simulink model "NMPC_BGLOSA_2VEH"  (R2022b)
settings: Solver=ode4  StartTime=0.0  StopTime=1500  FixedStep=0.1  RelTol=1e-3
PostLoadFcn:
  | , if any(exist('dsrtsu_mdlpostloadfcn', 'file') == [2, 3, 6]), try dsrtsu_mdlpostloadfcn('Execute', bdroot); catch fprintf('Error in PostLoadFcn (dsrtsu_mdlpostloadfcn) for model "%s":\n %s\n', bdroot, lasterr); end, end,
values from neighbouring files (symbols this model uses):
  k_road_map = k_road_map(:)    [NMPC_init_2veh.m]
  N = 50    [ACADO_2veh.m]    (also in NMPC_init_2veh.m; debug_vincoli_violati.m)
  N_iter = 3    [NMPC_init_2veh.m]
  N_Jterms = length(Qx1)    [NMPC_init_2veh.m]
  NMPC_Wmat1 = [W1(1,:) W1(2,:) W1(3,:) W1(4,:) W1(5,:) W1(6,:) W1(7,:) W1(8,:) W1(9,:) W1(10,:) W1(11,:) W1(12,:) W1(13,:) W1(14,:)]    [NMPC_init_2veh.m]
  NMPC_WNmat1 = reshape(WN1.',1,[])    [NMPC_init_2veh.m]
  t_dwell = 10    [ACADO_2veh.m]    (also in NMPC_init_2veh.m)
  t_offset = 0    [NMPC_init_2veh.m]
  time_bag_sim = (0:1:round(time_bag(end))-1)'    [NMPC_init_2veh.m]
  tl_state_sim = zeros(round(time_bag(end))-1,size(tl_col,2))    [NMPC_init_2veh.m]
  Ts = 1    [ACADO_2veh.m]    (also in NMPC_init_2veh.m)
  Vmax = 50    [NMPC_init_2veh.m]    (also in debug_vincoli_violati.m = OD(:,17))
  xInit = [20 2 0 0 1 0]    [NMPC_init_2veh.m]
undefined symbols (not defined in the file or in its folder): ds, s_start
libraries: simulink x1
(part 2 of 2)

== matlab function NMPC_BGLOSA_2VEH/NMPC WITH MOTOR DYNAMICS/ROAD PREVIEW/No ROAD PREVIEW ==
  data: x_TL input; stop_enabled input; Vmax input; Vmax_2 input; state_pred_old input; t_dwell input; time_cur input; reached_TL_old input; reached_TL_old_2 input; reached_stop_old input; reached_stop_old_2 input; t_piola_old input; t_loreto_old input; stop_dwell_count_old input; stop_dwell_count_old_2 input; OnlineData output; reached_TL output; reached_TL_2 output; reached_stop output; reached_stop_2 output; t_piola output; t_loreto output; debug_TL output; debug_TL_2 output; stop_dwell_count output; stop_dwell_count_2 output; red_stopline_hold output; s_hold output; k_road_hor input; red_stopline_hold2 output; s_hold2 output; k_road_hor_2 input
function [OnlineData, reached_TL, reached_TL_2, reached_stop, reached_stop_2, t_piola, t_loreto, debug_TL, debug_TL_2, stop_dwell_count, stop_dwell_count_2, red_stopline_hold, s_hold, red_stopline_hold2, s_hold2] = OnlineDataArray( x_TL, stop_enabled, Vmax, Vmax_2,state_pred_old,t_dwell, time_cur,reached_TL_old, reached_TL_old_2,reached_stop_old, reached_stop_old_2,t_piola_old, t_loreto_old,stop_dwell_count_old, stop_dwell_count_old_2,k_road_hor, k_road_hor_2)
% ============================================================
% ONLINE DATA ARRAY FOR NMPC-BGLOSA WITH RIGID PLATOON
% with reached_TL memory
% ============================================================
%
% OnlineData structure per prediction node(50):
%
%   1  - 11   x_TL_head
%   12        s_stop_active
%   13        x_stop_active
%   14        x_dwell_active
%   15        w_stop_active
%   16        k_road
%   17        Vmax
%   18        dt_schd
%   19        s_st
%   20        s_hor
%   21 - 31   x_TL_tail
%
%   32 - 42   x_TL_head_2
%   43        s_stop_active_2
%   44        x_stop_active_2
%   45        x_dwell_active_2
%   46        w_stop_active_2
%   47        k_road_2
%   48        Vmax_2
%   49        dt_schd_2
%   50        s_st_2
%   51        s_hor_2
%   52 - 62   x_TL_tail_2
%
%======convenzioni=============================================
%
% x_TL = 1  -> green / constraint released
% x_TL = 0  -> red / constraint active
%
% x_stop  = 1 -> vincolo di approccio rilasciato
% x_stop  = 0 -> vincolo di approccio attivo: pos <= s_stop
%
% x_dwell = 1 -> dwell attivo: stop-box attiva
% x_dwell = 0 -> dwell non attivo
%
% w_stop  = 1 -> costo di attrazione verso fermata attivo
% w_stop  = 0 -> costo di attrazione spento
%
%=============================================================
% ============================================================
% CONSTANTS
% ============================================================
N_od    = 62;
N_tl    = 11;
N_stops = 7;
N       = 50;
% ============================================================
% OnlineData indices
% ============================================================
% 1  - 11 : x_TL_head
idx_sstop_active  = 12;
idx_xstop_active  = 13;
idx_xdwell_active = 14;
idx_wstop_active  = 15;
idx_kroad         = 16;
idx_vmax          = 17;
idx_dtschd        = 18;
idx_sst           = 19;
idx_shor          = 20;
idx_tail0         = 20;  % 21 - 31 : x_TL_tail

idx_head0_2=31;
idx_sstop_active_2  = 43;
idx_xstop_active_2  = 44;
idx_xdwell_active_2 = 45;
idx_wstop_active_2  = 46;
idx_kroad_2         = 47;
idx_vmax_2          = 48;
idx_dtschd_2        = 49;
idx_sst_2           = 50;
idx_shor_2          = 51;
idx_tail0_2         = 51;  % 52 - 62 : x_TL_tail


L_platoon = 10;  % [m]


s_TL = [45.5, 203.2, 384.2, 589.4, 773.6, 1004.2,1225.3, 1419.7, 1507.8, 1739.0, 1823.0];
s_stop = [80, 447, 756, 1084, 1304, 1507, 1822];
s_max = 5200;
dt_schd_default = 180;
s_st_default    = 1e5;
s_hor_default   = 300;
debug_TL = zeros(N_tl,26);
debug_TL_2 = zeros(N_tl,26);
Ts = 1.0;
N_dwell_steps = max(1, round(t_dwell/Ts));


eps_stop_dwell = 0.8;   % [m]
eps_vel_dwell  = 0.05;  % [m/s]


% ============================================================
% DEBUG INITIALIZATION
% ============================================================
%
% debug_TL is kept with the same size as before to avoid breaking
% downstream scopes/displays. Its columns can later be redefined.
% ============================================================
% FIXED-SIZE OUTPUT INITIALIZATION
% ============================================================

OnlineData = zeros(N_od*(N+1),1);
reached_TL   = reached_TL_old;
reached_TL_2   = reached_TL_old_2;

t_piola      = t_piola_old;
t_loreto     = t_loreto_old;

reached_stop     = reached_stop_old;
reached_stop_2   = reached_stop_old_2;

stop_dwell_count = stop_dwell_count_old;
stop_dwell_count_2 = stop_dwell_count_old_2;

red_stopline_hold = 0.0;
s_hold            = 0.0;
red_stopline_hold2 = 0.0;
s_hold2            = 0.0;
% ============================================================
% PREDICTED STATES
% ============================================================

pos_hor      = state_pred_old(:,1);
vel_hor      = state_pred_old(:,2);
pos_hor_tail = pos_hor - L_platoon;

s_now = pos_hor(1);
v_now = vel_hor(1);

pos_hor_2      = state_pred_old(:,4);
vel_hor_2       = state_pred_old(:,5);
pos_hor_tail_2  = pos_hor_2  - L_platoon;

s_now_2  = pos_hor_2 (1);
v_now_2  = vel_hor_2 (1);

% ============================================================
% INITIAL ONLINE DATA VECTOR
% ============================================================

base_node = zeros(N_od,1);

% Traffic lights released by default: head
base_node(1:11) = 1;

% Active stop released by default
base_node(idx_sstop_active)  = s_max;
base_node(idx_xstop_active)  = 1;
base_node(idx_xdwell_active) = 0;
base_node(idx_wstop_active)  = 0;

% Road / speed / schedule
base_node(idx_kroad)  = 0;
base_node(idx_vmax)   = Vmax;
base_node(idx_dtschd) = dt_schd_default;
base_node(idx_sst)    = s_st_default;
base_node(idx_shor)   = s_hor_default;

% Traffic lights released by default: tail
base_node(21:31) = 1;




% Traffic lights released by default: head
base_node(32:42) = 1;

% Active stop released by default
base_node(idx_sstop_active_2)  = s_max;
base_node(idx_xstop_active_2)  = 1;
base_node(idx_xdwell_active_2) = 0;
base_node(idx_wstop_active_2)  = 0;

% Road / speed / schedule
base_node(idx_kroad_2)  = 0;
base_node(idx_vmax_2)   = Vmax_2;
base_node(idx_dtschd_2) = dt_schd_default;
base_node(idx_sst_2)    = s_st_default;
base_node(idx_shor_2)   = s_hor_default;

% Traffic lights released by default: tail
base_node(52:62) = 1;


% Replicate base node on whole horizon
for kk = 1:N+1
    idx0 = N_od*(kk-1);
    OnlineData(idx0+1:idx0+N_od) = base_node;
end



% ============================================================
% ROAD CURVATURE ONLINE DATA
% ============================================================
if numel(k_road_hor) == 1

    for kk = 1:N+1
        OnlineData(idx_kroad + N_od*(kk-1)) = abs(k_road_hor);
    end

else

    for kk = 1:N+1
        OnlineData(idx_kroad + N_od*(kk-1)) = abs(k_road_hor(kk));
    end

end
% ============================================================
% ROAD CURVATURE ONLINE DATA 2 VEH
% ============================================================
if numel(k_road_hor_2) == 1

    for kk = 1:N+1
        OnlineData(idx_kroad_2 + N_od*(kk-1)) = abs(k_road_hor_2);
    end

else

    for kk = 1:N+1
        OnlineData(idx_kroad_2 + N_od*(kk-1)) = abs(k_road_hor_2(kk));
    end

end



% ============================================================
% BUS STOP ONLINE DATA - SINGLE ACTIVE STOP FORMULATION
% ============================================================
%
% Only one stop is passed to ACADO:
%
%   s_stop_active
%   x_stop_active
%   x_dwell_active
%   w_stop_active
%
% Convention:
%
%   x_stop_active  = 0 -> approach constraint active: pos <= s_stop_active
%   x_stop_active  = 1 -> approach constraint released
%
%   x_dwell_active = 1 -> dwell stop-box active
%   x_dwell_active = 0 -> dwell inactive
%
%   w_stop_active  = 1 -> attraction cost toward stop active
%   w_stop_active  = 0 -> cost disabled
% ============================================================

stop_in_dwell_now = zeros(1,N_stops);

% ============================================================
% Saturate already completed stops
% ============================================================

for jj = 1:N_stops

    if reached_stop(jj) == 1
        stop_dwell_count(jj) = N_dwell_steps;
        stop_in_dwell_now(jj) = 0;
    end

end

% ============================================================
% Select first enabled and not completed stop
% ============================================================

active_stop_idx = 0;

for jj = 1:N_stops

    if reached_stop(jj) == 0 && stop_enabled(jj) == 1
        active_stop_idx = jj;
        break
    end

end

% ============================================================
% Update memory only for active stop
% ============================================================

if active_stop_idx > 0

    jj = active_stop_idx;
    s_bus_stop = s_stop(jj);

    bus_at_stop = abs(s_now - s_bus_stop) <= eps_stop_dwell && ...
                  abs(v_now) <= eps_vel_dwell;

    bus_passed_stop = s_now >= s_bus_stop + eps_stop_dwell;

    dwell_latched = stop_dwell_count(jj) > 0 && ...
                    stop_dwell_count(jj) < N_dwell_steps && ...
                    reached_stop(jj) == 0;

    if dwell_latched

        stop_in_dwell_now(jj) = 1;
        stop_dwell_count(jj) = stop_dwell_count(jj) + 1;

        if stop_dwell_count(jj) >= N_dwell_steps
            reached_stop(jj) = 1;
            stop_dwell_count(jj) = N_dwell_steps;
            stop_in_dwell_now(jj) = 0;
        end

    elseif bus_at_stop

        stop_in_dwell_now(jj) = 1;
        stop_dwell_count(jj) = 1;

        if stop_dwell_count(jj) >= N_dwell_steps
            reached_stop(jj) = 1;
            stop_dwell_count(jj) = N_dwell_steps;
            stop_in_dwell_now(jj) = 0;
        end

    elseif bus_passed_stop

        % Safety fallback: should not happen if the hard stop constraint works.
        reached_stop(jj) = 1;
        stop_dwell_count(jj) = N_dwell_steps;
        stop_in_dwell_now(jj) = 0;

    else

        stop_in_dwell_now(jj) = 0;

    end
end

% ============================================================
% Recompute next active stop after memory update
% ============================================================

next_stop_idx = 0;

for jj = 1:N_stops

    if reached_stop(jj) == 0 && stop_enabled(jj) == 1
        next_stop_idx = jj;
        break
    end

end

% ============================================================
% Write active stop OnlineData
% ============================================================
% Node kk = 1 remains released because the current state is fixed.
% Stop constraints are imposed from kk = 2.
% ============================================================

if next_stop_idx > 0

    jj = next_stop_idx;
    s_active = s_stop(jj);

    dwell_remaining = N_dwell_steps - stop_dwell_count(jj);

    if dwell_remaining < 0
        dwell_remaining = 0;
    end

    for kk = 2:N+1

        idx0 = N_od*(kk-1);

        OnlineData(idx0 + idx_sstop_active) = s_active;

        if stop_in_dwell_now(jj) == 1

            % DWELL_STOP:
            % Approach released, dwell active only for remaining dwell nodes.
            OnlineData(idx0 + idx_xstop_active) = 1;
            OnlineData(idx0 + idx_wstop_active) = 0;

            if kk <= dwell_remaining + 1
                OnlineData(idx0 + idx_xdwell_active) = 1;
            else
                OnlineData(idx0 + idx_xdwell_active) = 0;
            end

        else

            % APPROACH_STOP:
            % Approach constraint active and attraction cost enabled.
            OnlineData(idx0 + idx_xstop_active)  = 0;
            OnlineData(idx0 + idx_xdwell_active) = 0;
            OnlineData(idx0 + idx_wstop_active)  = 1;

        end
    end
end


% ============================================================
% BUS STOP ONLINE DATA - SINGLE ACTIVE STOP FORMULATION - 2 VEH
% ============================================================
%
% Second vehicle OnlineData indices:
%
%   43   s_stop_active_2
%   44   x_stop_active_2
%   45   x_dwell_active_2
%   46   w_stop_active_2
%
% Convention:
%
%   x_stop_active_2  = 0 -> approach constraint active: pos2 <= s_stop_active_2
%   x_stop_active_2  = 1 -> approach constraint released
%
%   x_dwell_active_2 = 1 -> dwell stop-box active
%   x_dwell_active_2 = 0 -> dwell inactive
%
%   w_stop_active_2  = 1 -> attraction cost toward active stop
%   w_stop_active_2  = 0 -> cost disabled
% ============================================================

stop_in_dwell_now_2 = zeros(1,N_stops);

% ============================================================
% Saturate already completed stops - vehicle 2
% ============================================================

for jj = 1:N_stops

    if reached_stop_2(jj) == 1
        stop_dwell_count_2(jj) = N_dwell_steps;
        stop_in_dwell_now_2(jj) = 0;
    end

end

% ============================================================
% Select first enabled and not completed stop - vehicle 2
% ============================================================

active_stop_idx_2 = 0;

for jj = 1:N_stops

    if reached_stop_2(jj) == 0 && stop_enabled(jj) == 1
        active_stop_idx_2 = jj;
        break
    end

end

% ============================================================
% Update memory only for active stop - vehicle 2
% ============================================================

if active_stop_idx_2 > 0

    jj = active_stop_idx_2;
    s_bus_stop_2 = s_stop(jj);

    bus_at_stop_2 = abs(s_now_2 - s_bus_stop_2) <= eps_stop_dwell && ...
                    abs(v_now_2) <= eps_vel_dwell;

    bus_passed_stop_2 = s_now_2 >= s_bus_stop_2 + eps_stop_dwell;

    dwell_latched_2 = stop_dwell_count_2(jj) > 0 && ...
                      stop_dwell_count_2(jj) < N_dwell_steps && ...
                      reached_stop_2(jj) == 0;

    if dwell_latched_2

        stop_in_dwell_now_2(jj) = 1;
        stop_dwell_count_2(jj) = stop_dwell_count_2(jj) + 1;

        if stop_dwell_count_2(jj) >= N_dwell_steps
            reached_stop_2(jj) = 1;
            stop_dwell_count_2(jj) = N_dwell_steps;
            stop_in_dwell_now_2(jj) = 0;
        end

    elseif bus_at_stop_2

        stop_in_dwell_now_2(jj) = 1;
        stop_dwell_count_2(jj) = 1;

        if stop_dwell_count_2(jj) >= N_dwell_steps
            reached_stop_2(jj) = 1;
            stop_dwell_count_2(jj) = N_dwell_steps;
            stop_in_dwell_now_2(jj) = 0;
        end

    elseif bus_passed_stop_2

        % Safety fallback: should not happen if the hard stop constraint works.
        reached_stop_2(jj) = 1;
        stop_dwell_count_2(jj) = N_dwell_steps;
        stop_in_dwell_now_2(jj) = 0;

    else

        stop_in_dwell_now_2(jj) = 0;

    end

end

% ============================================================
% Recompute next active stop after memory update - vehicle 2
% ============================================================

next_stop_idx_2 = 0;

for jj = 1:N_stops

    if reached_stop_2(jj) == 0 && stop_enabled(jj) == 1
        next_stop_idx_2 = jj;
        break
    end

end

% ============================================================
% Write active stop OnlineData - vehicle 2
% ============================================================
% Node kk = 1 remains released because the current state is fixed.
% Stop constraints are imposed from kk = 2.
% ============================================================

if next_stop_idx_2 > 0

    jj = next_stop_idx_2;
    s_active_2 = s_stop(jj);

    dwell_remaining_2 = N_dwell_steps - stop_dwell_count_2(jj);

    if dwell_remaining_2 < 0
        dwell_remaining_2 = 0;
    end

    for kk = 2:N+1

        idx0 = N_od*(kk-1);

        OnlineData(idx0 + idx_sstop_active_2) = s_active_2;

        if stop_in_dwell_now_2(jj) == 1

            % DWELL_STOP:
            % Approach released, dwell active only for remaining dwell nodes.
            OnlineData(idx0 + idx_xstop_active_2) = 1;
            OnlineData(idx0 + idx_wstop_active_2) = 0;

            if kk <= dwell_remaining_2 + 1
                OnlineData(idx0 + idx_xdwell_active_2) = 1;
            else
                OnlineData(idx0 + idx_xdwell_active_2) = 0;
            end

        else

            % APPROACH_STOP:
            % Approach constraint active and attraction cost enabled.
            OnlineData(idx0 + idx_xstop_active_2)  = 0;
            OnlineData(idx0 + idx_xdwell_active_2) = 0;
            OnlineData(idx0 + idx_wstop_active_2)  = 1;

        end

    end

end


%=============================================================
% TRAFFIC LIGHT ONLINE DATA: aggiornamento vincoli testa/coda
% con memoria dei semafori già raggiunti
% ============================================================
%
% Per ogni step corrente si scorre su tutti i semafori e si aggiornano
% i flag dei vincoli per testa e coda del platoon.
%
% Convenzione:
%   x_TL = 1  -> verde / vincolo rilasciato
%   x_TL = 0  -> rosso / vincolo attivo
%
% Il nodo kk = 1 rappresenta lo stato corrente già fissato dal plant.
% Per questo motivo i vincoli semaforici vengono applicati solo da kk = 2.
%
% Nota importante:
%   Il crossing corrente della testa/coda NON deve usare il margine di
%   clearing della coda.
%
%   Sono introdotte tre soglie distinte:
%
%   eps_cross_now:
%       soglia piccola per decidere se al nodo corrente testa/coda sono
%       già oltre la stop-line.
%
%   eps_clear_tail:
%       margine fisico più grande usato solo per verificare se la coda
%       ha liberato robustamente il TL entro la fine del verde.
%
%   eps_stopline_commit:
%       fascia numerica molto stretta attorno alla stop-line. Se il veicolo
%       è praticamente fermo in questa fascia, non si impone più un vincolo
%       rosso hard, perché il problema diventa numericamente fragile.
% ============================================================

for ii = 1:N_tl

    % ========================================================
    % DEBUG CLASSIFICATION: significato di main_case
    % ========================================================
    %
    % main_case:
    %
    % 1 = TL già superato al nodo corrente.
    %     Si entra in questo caso solo se testa o coda sono realmente oltre
    %     la linea semaforica, oppure se reached_TL_old(ii) è già attivo.
    %
    % 2 = Copia base dello SPaT sull'orizzonte predittivo.
    %
    % 3 = Verde corrente liberabile dalla coda secondo state_pred_old.
    %
    % 4 = La testa non raggiunge il TL nell'orizzonte.
    %
    % 5 = La testa raggiunge il TL, ma la coda non lo libera nell'orizzonte.
    %
    % 6 = Testa e coda attraversano nella stessa finestra verde valida.
    %
    % 7 = Attraversamento previsto, ma senza finestra verde comune valida.
    % 7A(7.3)=commitment stop-line verde
    % 7B(7.6)=blocco in ingresso a stop-line
    % 7C(11)=caso critico, blocco non catturato
    %
    % 8 = Fallback cinematico positivo.
    %
    % 9 = Verde corrente non liberabile dalla coda.
    %     Se il veicolo è fermo sulla stop-line e il TL è verde, viene
    %     applicato il commitment: testa e coda vengono rilasciate.
    %9A(9)=commitmenti stop-line su verde
    %9B(9.3)=blocco su stop-line
    %9C(10)=blocco non catturato
    %
    % mem_case:
    %
    % 0 = nessun aggiornamento di memoria.
    % 1 = coda già oltre il TL.
    % 2 = testa già oltre il TL.
    % 3 = testa ferma sulla linea, ma non ancora oltre.
    % 4 = non ancora utilizzato
    % ========================================================

    main_case = 0;
    mem_case  = 0;

    % ========================================================
    % INIZIALIZZAZIONE VARIABILI LOCALI DEL SEMAFORO ii
    % ========================================================

    current_green_end = 0;
    i_head_cross      = 0;
    i_tail_cross      = 0;
    green_window_ok   = 0;
    tail_at_green_end = -1e6;

%     green_start = 0;
%     green_end   = 0;
% 
%     release_head_from = 0;
%     release_tail_from = 0;

    s_light = s_TL(ii);

    % ========================================================
    % PARAMETRI NUMERICI LOCALI
    % ========================================================
    
    % Soglie fisiche, non numeriche
    eps_cross_head      = 0.05;   % [m] testa realmente oltre TL
    eps_cross_tail      = 0.20;   % [m] coda realmente oltre TL
    eps_clear_tail      = 0.20;   % [m] clearing robusto della coda
    eps_cross_now=eps_cross_head;
    
    % Fascia di stop-line
    d_stopline_deadband = 0.30;   % [m]
    v_deadband          = 0.02;   % [m/s]
    
    % Soglie già presenti
    a_brake_guard       = 1.5;    % [m/s^2]
    d_margin_guard      = 0.20;   % [m]
    v_stop_thr_guard    = 0.20;   % [m/s]
    
    eps_line            = 0.30;   % [m]

    % ========================================================
    % CLASSIFICAZIONE DELLO STATO CORRENTE RISPETTO ALLA STOP-LINE
    % ========================================================

    d_avail_now      = s_light - pos_hor(1);
    d_avail_tail_now = s_light - pos_hor_tail(1);
    
    % Crossing robusto: non usare 1e-6 m
    head_crossed_now = d_avail_now      < -eps_cross_head;
    tail_crossed_now = d_avail_tail_now < -eps_cross_tail;
    
    % Veicolo fermo sulla stop-line
    head_stopped_at_light = ...
        abs(d_avail_now) <= d_stopline_deadband && ...
        abs(vel_hor(1)) <= v_deadband && ...
        ~head_crossed_now;
    
    % Caso specifico: fermo sulla stop-line con semaforo rosso
    head_stopped_at_red = x_TL(1,ii) == 0 && head_stopped_at_light;


    % ========================================================
    % DEFAULT MEMORY PROPAGATION
    % ========================================================

    reached_TL(ii) = reached_TL_old(ii);

    % ========================================================
    % CASE 1 DA MEMORIA - TL già raggiunto in uno step precedente
    % ========================================================

    if reached_TL_old(ii) == 1

        for kk = 1:N+1
            idx_head = ii + N_od*(kk-1);
            idx_tail = idx_tail0 + ii + N_od*(kk-1);

            OnlineData(idx_head) = 1;
            OnlineData(idx_tail) = 1;
        end

        reached_TL(ii) = 1;
        main_case = 1;


        debug_TL(ii,:) = local_debug_row(time_cur, ii, s_light,pos_hor, pos_hor_tail, vel_hor,reached_TL_old, reached_TL, x_TL, OnlineData,N_od, idx_tail0,head_crossed_now, tail_crossed_now, head_stopped_at_light,mem_case, main_case, current_green_end,i_head_cross, i_tail_cross, green_window_ok, tail_at_green_end);
        continue
    end

    % ========================================================
    % MEMORY UPDATE
    % ========================================================

    if tail_crossed_now

        reached_TL(ii) = 1;
        mem_case = 1;

    elseif head_crossed_now

        reached_TL(ii) = 1;
        mem_case = 2;

    elseif head_stopped_at_light

        reached_TL(ii) = 0;
        mem_case = 3;

    else

        reached_TL(ii) = 0;
        mem_case = 0;

    end

    % ========================================================
    % CASE 1 - TL già superato al nodo corrente
    % ========================================================

    if head_crossed_now || tail_crossed_now

        for kk = 1:N+1
            idx_head = ii + N_od*(kk-1);
            idx_tail = idx_tail0 + ii + N_od*(kk-1);

            OnlineData(idx_head) = 1;
            OnlineData(idx_tail) = 1;
        end

        reached_TL(ii) = 1;
        main_case = 1;

        debug_TL(ii,:) = local_debug_row(time_cur, ii, s_light,pos_hor, pos_hor_tail, vel_hor,reached_TL_old, reached_TL, x_TL, OnlineData,N_od, idx_tail0,head_crossed_now, tail_crossed_now, head_stopped_at_light,mem_case, main_case, current_green_end,i_head_cross, i_tail_cross, green_window_ok, tail_at_green_end);

        continue
    end

    % ========================================================
    % CASE 2 - Copia base dello SPaT sull'orizzonte predittivo
    % ========================================================

    OnlineData(ii)             = 1;
    OnlineData(idx_tail0 + ii) = 1;

    for kk = 2:N+1
        idx_head = ii + N_od*(kk-1);
        idx_tail = idx_tail0 + ii + N_od*(kk-1);

        OnlineData(idx_head) = x_TL(kk,ii);
        OnlineData(idx_tail) = x_TL(kk,ii);
    end

    main_case = 2;
    % ========================================================
    % CASE 2B - STOP-LINE RED HOLD
    % ========================================================
    %
    % Il veicolo è praticamente fermo sulla stop-line mentre il TL è rosso.
    % Non dichiaro il TL superato.
    % Non rilascio il vincolo.
    % Mantengo x_TL = 0 finché il semaforo resta rosso.
    %
    % Questo evita che piccoli attraversamenti numerici vengano interpretati
    % come superamento reale del semaforo.
    % ========================================================
    
    if head_stopped_at_red
        red_stopline_hold = 1;
        s_hold = s_light;
    
        reached_TL(ii) = 0;
        mem_case = 3;
    
        for kk = 2:N+1
            idx_head = ii + N_od*(kk-1);
            idx_tail = idx_tail0 + ii + N_od*(kk-1);
    
            OnlineData(idx_head) = 0;
            OnlineData(idx_tail) = 0;
        end
    
        main_case = 5.5;
    
        debug_TL(ii,:) = local_debug_row( ...
            time_cur, ii, s_light, ...
            pos_hor, pos_hor_tail, vel_hor, ...
            reached_TL_old, reached_TL, x_TL, OnlineData, ...
            N_od, idx_tail0, ...
            head_crossed_now, tail_crossed_now, head_stopped_at_light, ...
            mem_case, main_case, current_green_end, ...
            i_head_cross, i_tail_cross, green_window_ok, tail_at_green_end);
    
        continue
    end

    % ========================================================
    % CASE 3 - Verde corrente liberabile dalla coda secondo state_pred_old
    % ========================================================

    if x_TL(1,ii) == 1

        current_green_end = local_current_green_end(x_TL, ii, N);

        if current_green_end > 0

            tail_at_green_end = pos_hor_tail(current_green_end);

            if tail_at_green_end > s_light + eps_clear_tail

                for kk = 1:N+1
                    idx_head = ii + N_od*(kk-1);
                    idx_tail = idx_tail0 + ii + N_od*(kk-1);

                    OnlineData(idx_head) = 1;
                    OnlineData(idx_tail) = 1;
                end

                main_case = 3;
                debug_TL(ii,:) = local_debug_row(time_cur, ii, s_light,pos_hor, pos_hor_tail, vel_hor,reached_TL_old, reached_TL, x_TL, OnlineData,N_od, idx_tail0,head_crossed_now, tail_crossed_now, head_stopped_at_light,mem_case, main_case, current_green_end,i_head_cross, i_tail_cross, green_window_ok, tail_at_green_end);

                continue
            end
        end
    end

% ========================================================
% CASE 4 - Testa non raggiunge il TL nell'orizzonte
% ========================================================

    i_head_cross = 0;
    i_tail_cross = 0;
    
    for kk = 2:N+1
        if pos_hor(kk) >= s_light
            i_head_cross = kk;
            break
        end
    end
    
    if i_head_cross == 0
    
        main_case = 4;
    
        debug_TL(ii,:) = local_debug_row( ...
            time_cur, ii, s_light, ...
            pos_hor, pos_hor_tail, vel_hor, ...
            reached_TL_old, reached_TL, x_TL, OnlineData, ...
            N_od, idx_tail0, ...
            head_crossed_now, tail_crossed_now, head_stopped_at_light, ...
            mem_case, main_case, current_green_end, ...
            i_head_cross, i_tail_cross, green_window_ok, tail_at_green_end);
    
        continue
    end
    
    % ========================================================
    % CASE 5 / 8 / 9 - Testa raggiunge il TL, coda non necessariamente
    %                  liberante nell'orizzonte
    % ========================================================
    
    for kk = 2:N+1
        if pos_hor_tail(kk) >= s_light
            i_tail_cross = kk;
            break
        end
    end

    if i_tail_cross == 0

        main_case = 5;

        % ====================================================
        % Se il TL è verde al nodo corrente, valuto case 8/9.
        % ====================================================

        if x_TL(1,ii) == 1

            current_green_end = local_current_green_end(x_TL, ii, N);

            if current_green_end > 0

                tail_at_green_end = pos_hor_tail(current_green_end);

                % ====================================================
                % Stima cinematica conservativa del clearing della coda
                % ====================================================

                dist_tail_to_TL = s_light - pos_hor_tail(1);

                if dist_tail_to_TL < 0
                    dist_tail_to_TL = 0;
                end

                v0_clear = vel_hor(1);
                if v0_clear < 0
                    v0_clear = 0;
                end

                a_clear     = 0.7;   % [m/s^2]
                v_max_clear = Vmax;  % [m/s]

                if dist_tail_to_TL <= 0
                    t_clear_tail = 0;

                else
                    
                    if v0_clear >= v_max_clear || a_clear <= 0
                        t_clear_tail = dist_tail_to_TL / max(v0_clear, 0.1);

                    else

                        t_to_vmax = (v_max_clear - v0_clear) / a_clear;
                        d_to_vmax = v0_clear*t_to_vmax + 0.5*a_clear*t_to_vmax^2;

                        if dist_tail_to_TL <= d_to_vmax

                            t_clear_tail =(-v0_clear + sqrt(v0_clear^2 + 2*a_clear*dist_tail_to_TL)) / a_clear;

                        else
                            t_clear_tail =t_to_vmax + (dist_tail_to_TL - d_to_vmax) / v_max_clear;
                        end
                    end
                end
                dt_pred = 1.0;
                kk_tail_clear_est = ceil(t_clear_tail/dt_pred) + 1;

                if kk_tail_clear_est < 2
                    kk_tail_clear_est = 2;
                end

                tail_margin_nodes = 1;

                % ====================================================
                % CASE 8 - Fallback cinematico positivo
                % ====================================================

                if kk_tail_clear_est + tail_margin_nodes <= current_green_end

                    for kk = 2:N+1
                        idx_head = ii + N_od*(kk-1);
                        idx_tail = idx_tail0 + ii + N_od*(kk-1);
                        OnlineData(idx_head) = 1;

                        if kk < kk_tail_clear_est
                            OnlineData(idx_tail) = 0;
                        else
                            OnlineData(idx_tail) = 1;
                        end
                    end

                    main_case       = 8;
                    green_window_ok = 1;

                    debug_TL(ii,:) = local_debug_row(time_cur, ii, s_light,pos_hor, pos_hor_tail, vel_hor,reached_TL_old, reached_TL, x_TL, OnlineData,N_od, idx_tail0,head_crossed_now, tail_crossed_now, head_stopped_at_light,mem_case, main_case, current_green_end,i_head_cross, i_tail_cross, green_window_ok, tail_at_green_end);

                    continue

                else

                    d_avail     = s_light - pos_hor(1);
                    d_stop_phys = vel_hor(1)^2/(2*a_brake_guard);

                    % =================================================
                    % CASE 9 - Verde corrente non liberabile dalla coda
                    % =================================================
                    %
                    % Commitment:
                    %   se il veicolo è fermo praticamente sulla stop-line
                    %   e il TL è verde, il veicolo viene autorizzato a
                    %   entrare e completare l'attraversamento.
                    %
                    %   Quindi si rilasciano sia testa sia coda.
                    %
                    %   Non si imposta reached_TL(ii)=1 qui: la memoria viene
                    %   aggiornata solo quando la testa o la coda superano
                    %   realmente la linea.
                    % =================================================

                    already_stopped_before_line =  (vel_hor(1) <= v_stop_thr_guard) && (d_avail >= 0);

                    can_still_stop =already_stopped_before_line || (d_avail >= d_stop_phys + d_margin_guard);

                    stopline_green_release =(x_TL(1,ii) == 1) && (d_avail >= 0) && (d_avail <= eps_line) && (vel_hor(1) <= v_stop_thr_guard);
                    
                    
                    if stopline_green_release
                    
                        % =================================================
                        % CASE 9A - GREEN COMMIT DA STOP-LINE
                        % =================================================
                        %
                        % Il veicolo era fermo sulla stop-line al rosso.
                        % Appena il TL diventa verde, viene autorizzato a partire.
                        %
                        % Da questo istante il TL viene marcato come "superato"
                        % dal punto di vista logico, così ai campioni successivi
                        % si entra direttamente nel CASE 1 da memoria.
                        % =================================================
                    
                        for kk_case9 = 1:N+1
                    
                            idx_head = ii + N_od*(kk_case9-1);
                            idx_tail = idx_tail0 + ii + N_od*(kk_case9-1);
                    
                            OnlineData(idx_head) = 1;
                            OnlineData(idx_tail) = 1;
                    
                        end
                    
                        reached_TL(ii) = 1;
                        mem_case       = 4;     % green commit
                        main_case      = 9;
                        green_window_ok = 1;
                    
                        debug_TL(ii,:) = local_debug_row( ...
                            time_cur, ii, s_light, ...
                            pos_hor, pos_hor_tail, vel_hor, ...
                            reached_TL_old, reached_TL, x_TL, OnlineData, ...
                            N_od, idx_tail0, ...
                            head_crossed_now, tail_crossed_now, head_stopped_at_light, ...
                            mem_case, main_case, current_green_end, ...
                            i_head_cross, i_tail_cross, green_window_ok, tail_at_green_end);
                    
                        continue

                    elseif can_still_stop || d_avail >= eps_line

                        % =================================================
                        % CASE 9B - Blocco ingresso
                        % =================================================
                        %
                        % Il veicolo è ancora chiaramente prima della linea.
                        % In questo caso il blocco ingresso è corretto.
                        % =================================================

                        for kk_case9 = 2:current_green_end
                            idx_head = ii + N_od*(kk_case9-1);
                            idx_tail = idx_tail0 + ii + N_od*(kk_case9-1);

                            OnlineData(idx_head) = 0;
                            OnlineData(idx_tail) = 0;
                        end

                        main_case = 9.3;
                        debug_TL(ii,:) = local_debug_row(time_cur, ii, s_light,pos_hor, pos_hor_tail, vel_hor,reached_TL_old, reached_TL, x_TL, OnlineData,N_od, idx_tail0,head_crossed_now, tail_crossed_now, head_stopped_at_light,mem_case, main_case, current_green_end,i_head_cross, i_tail_cross, green_window_ok, tail_at_green_end);


%                     else
% 
%                         % =================================================
%                         % CASE 9C - Stato già oltre la linea ma non catturato prima
%                         %non utilizzato
%                         % =================================================
% 
%                         for kk_case9 = 1:N+1
%                             idx_head = ii + N_od*(kk_case9-1);
%                             idx_tail = idx_tail0 + ii + N_od*(kk_case9-1);
% 
%                             OnlineData(idx_head) = 1;
%                             OnlineData(idx_tail) = 1;
%                         end
% 
%                         reached_TL(ii) = 1;
%                         main_case = 10;
%                         mem_case  = 2;
% 
                     end

                    green_window_ok = 0;

                    debug_TL(ii,:) = local_debug_row(time_cur, ii, s_light,pos_hor, pos_hor_tail, vel_hor,reached_TL_old, reached_TL, x_TL, OnlineData,N_od, idx_tail0,head_crossed_now, tail_crossed_now, head_stopped_at_light,mem_case, main_case, current_green_end,i_head_cross, i_tail_cross, green_window_ok, tail_at_green_end);

                    continue
                end
            end
        end

        % ====================================================
        % CASE 5 - Default con coda non attraversante
        % ====================================================

        d_avail = s_light - pos_hor(1);

        case5_crossed = d_avail < -eps_cross_now;

        if case5_crossed

            for kk_case5 = 1:N+1
                idx_head = ii + N_od*(kk_case5-1);
                idx_tail = idx_tail0 + ii + N_od*(kk_case5-1);

                OnlineData(idx_head) = 1;
                OnlineData(idx_tail) = 1;
            end

            reached_TL(ii) = 1;
            main_case = 10;
            mem_case  = 2;
        end
        debug_TL(ii,:) = local_debug_row(time_cur, ii, s_light,pos_hor, pos_hor_tail, vel_hor,reached_TL_old, reached_TL, x_TL, OnlineData,N_od, idx_tail0,head_crossed_now, tail_crossed_now, head_stopped_at_light,mem_case, main_case, current_green_end,i_head_cross, i_tail_cross, green_window_ok, tail_at_green_end);

        continue
    end

    % ========================================================
    % Verifica della finestra verde comune per testa e coda
    % ========================================================

    green_info = local_find_green_window_vec(x_TL, ii, N, i_head_cross, i_tail_cross);

    green_window_ok = green_info(1);
    green_start = green_info(2);
    green_end = green_info(3);

    if green_window_ok == 1

        release_head_from = i_head_cross;
        release_tail_from = i_tail_cross;

        % ====================================================
        % Guard sulla transizione rosso-verde
        % ====================================================

        if green_start > 1
            if x_TL(green_start-1,ii) == 0 && x_TL(green_start,ii) == 1

                %release_head_from = max(release_head_from, green_start+2);
                release_head_from = max(release_head_from, green_start);
                release_tail_from = max(release_tail_from, green_start);

            end
        end

        if release_head_from > green_end || release_tail_from > green_end

            main_case       = 7;
            green_window_ok = 0;

        else

            % =================================================
            % CASE 6 - Attraversamento valido nella stessa finestra verde
            % =================================================

            for kk = 2:N+1

                idx_head = ii + N_od*(kk-1);
                idx_tail = idx_tail0 + ii + N_od*(kk-1);

                if kk < release_head_from
                    OnlineData(idx_head) = 0;
                else
                    OnlineData(idx_head) = 1;
                end

                if kk < release_tail_from
                    OnlineData(idx_tail) = 0;
                else
                    OnlineData(idx_tail) = 1;
                end
            end

            main_case = 6;
        end

    else

        main_case = 7;

    end

    % ========================================================
    % PROTEZIONE AGGIUNTIVA DEL CASE 7 SU VERDE CORRENTE
    % ========================================================

    if main_case == 7 && x_TL(1,ii) == 1

        current_green_end = local_current_green_end(x_TL, ii, N);

        if current_green_end > 0

            d_avail     = s_light - pos_hor(1);
            d_stop_phys = vel_hor(1)^2/(2*a_brake_guard);

            already_stopped_before_line =(vel_hor(1) <= v_stop_thr_guard) && (d_avail >= 0);

            can_still_stop = already_stopped_before_line ||(d_avail >= d_stop_phys + d_margin_guard);

            stopline_green_release = (x_TL(1,ii) == 1) && (d_avail >= 0) && (d_avail <= eps_line) && (vel_hor(1) <= v_stop_thr_guard);

           if stopline_green_release

                % ====================================================
                % CASE 7A - GREEN COMMIT DA STOP-LINE
                % ====================================================
            
                for kk_case7 = 1:N+1
            
                    idx_head = ii + N_od*(kk_case7-1);
                    idx_tail = idx_tail0 + ii + N_od*(kk_case7-1);
            
                    OnlineData(idx_head) = 1;
                    OnlineData(idx_tail) = 1;
            
                end
            
                reached_TL(ii) = 1;
                mem_case       = 4;     % green commit
                main_case      = 7.3;
                green_window_ok = 1;
         
            elseif can_still_stop || d_avail >= eps_line

                % ====================================================
                % CASE 7B - Blocco ingresso (7.6)
                % ====================================================

                for kk_case7 = 2:current_green_end
                    idx_head = ii + N_od*(kk_case7-1);
                    idx_tail = idx_tail0 + ii + N_od*(kk_case7-1);
                    OnlineData(idx_head) = 0;
                    OnlineData(idx_tail) = 0;
                end

                green_window_ok = 0;
                main_case=7.6;

%             else
% 
%                 % ====================================================
%                 % CASE 7C - Stato già oltre la linea ma non catturato prima
%                 % non utilizzato
%                 % ====================================================
% 
%                 for kk_case7 = 1:N+1
%                     idx_head = ii + N_od*(kk_case7-1);
%                     idx_tail = idx_tail0 + ii + N_od*(kk_case7-1);
% 
%                     OnlineData(idx_head) = 1;
%                     OnlineData(idx_tail) = 1;
%                 end
% 
%                 reached_TL(ii) = 1;
%                 main_case = 11;
%                 mem_case  = 2;
%                 green_window_ok = 0;
% 
             end
        end
    end

    % ========================================================
    % DEBUG FINALE DEL SEMAFORO ii
    % ========================================================

    debug_TL(ii,:) = local_debug_row(time_cur, ii, s_light,pos_hor, pos_hor_tail, vel_hor,reached_TL_old, reached_TL, x_TL, OnlineData,N_od, idx_tail0,head_crossed_now, tail_crossed_now, head_stopped_at_light,mem_case, main_case, current_green_end,i_head_cross, i_tail_cross, green_window_ok, tail_at_green_end);
end



% ============================================================
% TRAFFIC LIGHT ONLINE DATA - 2 VEH
% aggiornamento vincoli testa/coda del secondo veicolo
% con memoria dei semafori già raggiunti
% ============================================================

for ii = 1:N_tl

    main_case = 0;
    mem_case  = 0;

    current_green_end = 0;
    i_head_cross      = 0;
    i_tail_cross      = 0;
    green_window_ok   = 0;
    tail_at_green_end = -1e6;

    s_light = s_TL(ii);

    % ========================================================
    % PARAMETRI NUMERICI LOCALI
    % ========================================================

    eps_cross_head      = 0.05;   % [m]
    eps_cross_tail      = 0.20;   % [m]
    eps_clear_tail      = 0.20;   % [m]
    eps_cross_now       = eps_cross_head;

    d_stopline_deadband = 0.30;   % [m]
    v_deadband          = 0.02;   % [m/s]

    a_brake_guard       = 1.5;    % [m/s^2]
    d_margin_guard      = 0.20;   % [m]
    v_stop_thr_guard    = 0.20;   % [m/s]

    eps_line            = 0.30;   % [m]

    % ========================================================
    % CLASSIFICAZIONE STATO CORRENTE VEICOLO 2
    % ========================================================

    d_avail_now_2      = s_light - pos_hor_2(1);
    d_avail_tail_now_2 = s_light - pos_hor_tail_2(1);

    head_crossed_now_2 = d_avail_now_2      < -eps_cross_head;
    tail_crossed_now_2 = d_avail_tail_now_2 < -eps_cross_tail;

    head_stopped_at_light_2 = ...
        abs(d_avail_now_2) <= d_stopline_deadband && ...
        abs(vel_hor_2(1)) <= v_deadband && ...
        ~head_crossed_now_2;

    head_stopped_at_red_2 = x_TL(1,ii) == 0 && head_stopped_at_light_2;

    % ========================================================
    % DEFAULT MEMORY PROPAGATION - VEH 2
    % ========================================================

    reached_TL_2(ii) = reached_TL_old_2(ii);

    % ========================================================
    % CASE 1 DA MEMORIA - TL già raggiunto in uno step precedente
    % ========================================================

    if reached_TL_old_2(ii) == 1

        for kk = 1:N+1

            idx_head = idx_head0_2 + ii + N_od*(kk-1);
            idx_tail = idx_tail0_2 + ii + N_od*(kk-1);

            OnlineData(idx_head) = 1;
            OnlineData(idx_tail) = 1;

        end

        reached_TL_2(ii) = 1;
        main_case = 1;

        debug_TL_2(ii,:) = local_debug_row_veh( ...
            time_cur, ii, s_light, ...
            pos_hor_2, pos_hor_tail_2, vel_hor_2, ...
            reached_TL_old_2, reached_TL_2, x_TL, OnlineData, ...
            N_od, idx_head0_2, idx_tail0_2, ...
            head_crossed_now_2, tail_crossed_now_2, head_stopped_at_light_2, ...
            mem_case, main_case, current_green_end, ...
            i_head_cross, i_tail_cross, green_window_ok, tail_at_green_end);

        continue

    end

    % ========================================================
    % MEMORY UPDATE - VEH 2
    % ========================================================

    if tail_crossed_now_2

        reached_TL_2(ii) = 1;
        mem_case = 1;

    elseif head_crossed_now_2

        reached_TL_2(ii) = 1;
        mem_case = 2;

    elseif head_stopped_at_light_2

        reached_TL_2(ii) = 0;
        mem_case = 3;

    else

        reached_TL_2(ii) = 0;
        mem_case = 0;

    end

    % ========================================================
    % CASE 1 - TL già superato al nodo corrente
    % ========================================================

    if head_crossed_now_2 || tail_crossed_now_2

        for kk = 1:N+1

            idx_head = idx_head0_2 + ii + N_od*(kk-1);
            idx_tail = idx_tail0_2 + ii + N_od*(kk-1);

            OnlineData(idx_head) = 1;
            OnlineData(idx_tail) = 1;

        end

        reached_TL_2(ii) = 1;
        main_case = 1;

        debug_TL_2(ii,:) = local_debug_row_veh( ...
            time_cur, ii, s_light, ...
            pos_hor_2, pos_hor_tail_2, vel_hor_2, ...
            reached_TL_old_2, reached_TL_2, x_TL, OnlineData, ...
            N_od, idx_head0_2, idx_tail0_2, ...
            head_crossed_now_2, tail_crossed_now_2, head_stopped_at_light_2, ...
            mem_case, main_case, current_green_end, ...
            i_head_cross, i_tail_cross, green_window_ok, tail_at_green_end);

        continue

    end

    % ========================================================
    % CASE 2 - Copia base dello SPaT sull'orizzonte predittivo
    % ========================================================

    OnlineData(idx_head0_2 + ii) = 1;
    OnlineData(idx_tail0_2 + ii) = 1;

    for kk = 2:N+1

        idx_head = idx_head0_2 + ii + N_od*(kk-1);
        idx_tail = idx_tail0_2 + ii + N_od*(kk-1);

        OnlineData(idx_head) = x_TL(kk,ii);
        OnlineData(idx_tail) = x_TL(kk,ii);

    end

    main_case = 2;

    % ========================================================
    % CASE 2B - STOP-LINE RED HOLD - VEH 2
    % ========================================================

    if head_stopped_at_red_2

        red_stopline_hold2 = 1;
        s_hold2 = s_light;

        reached_TL_2(ii) = 0;
        mem_case = 3;

        for kk = 2:N+1

            idx_head = idx_head0_2 + ii + N_od*(kk-1);
            idx_tail = idx_tail0_2 + ii + N_od*(kk-1);

            OnlineData(idx_head) = 0;
            OnlineData(idx_tail) = 0;

        end

        main_case = 5.5;

        debug_TL_2(ii,:) = local_debug_row_veh( ...
            time_cur, ii, s_light, ...
            pos_hor_2, pos_hor_tail_2, vel_hor_2, ...
            reached_TL_old_2, reached_TL_2, x_TL, OnlineData, ...
            N_od, idx_head0_2, idx_tail0_2, ...
            head_crossed_now_2, tail_crossed_now_2, head_stopped_at_light_2, ...
            mem_case, main_case, current_green_end, ...
            i_head_cross, i_tail_cross, green_window_ok, tail_at_green_end);

        continue

    end

    % ========================================================
    % CASE 3 - Verde corrente liberabile dalla coda - VEH 2
    % ========================================================

    if x_TL(1,ii) == 1

        current_green_end = local_current_green_end(x_TL, ii, N);

        if current_green_end > 0

            tail_at_green_end = pos_hor_tail_2(current_green_end);

            if tail_at_green_end > s_light + eps_clear_tail

                for kk = 1:N+1

                    idx_head = idx_head0_2 + ii + N_od*(kk-1);
                    idx_tail = idx_tail0_2 + ii + N_od*(kk-1);

                    OnlineData(idx_head) = 1;
                    OnlineData(idx_tail) = 1;

                end

                main_case = 3;

                debug_TL_2(ii,:) = local_debug_row_veh( ...
                    time_cur, ii, s_light, ...
                    pos_hor_2, pos_hor_tail_2, vel_hor_2, ...
                    reached_TL_old_2, reached_TL_2, x_TL, OnlineData, ...
                    N_od, idx_head0_2, idx_tail0_2, ...
                    head_crossed_now_2, tail_crossed_now_2, head_stopped_at_light_2, ...
                    mem_case, main_case, current_green_end, ...
                    i_head_cross, i_tail_cross, green_window_ok, tail_at_green_end);

                continue

            end

        end

    end

    % ========================================================
    % CASE 4 - Testa non raggiunge il TL nell'orizzonte - VEH 2
    % ========================================================

    i_head_cross = 0;
    i_tail_cross = 0;

    for kk = 2:N+1

        if pos_hor_2(kk) >= s_light
            i_head_cross = kk;
            break
        end

    end

    if i_head_cross == 0

        main_case = 4;

        debug_TL_2(ii,:) = local_debug_row_veh( ...
            time_cur, ii, s_light, ...
            pos_hor_2, pos_hor_tail_2, vel_hor_2, ...
            reached_TL_old_2, reached_TL_2, x_TL, OnlineData, ...
            N_od, idx_head0_2, idx_tail0_2, ...
            head_crossed_now_2, tail_crossed_now_2, head_stopped_at_light_2, ...
            mem_case, main_case, current_green_end, ...
            i_head_cross, i_tail_cross, green_window_ok, tail_at_green_end);

        continue

    end

    % ========================================================
    % CASE 5 / 8 / 9 - Testa raggiunge, coda non necessariamente
    %                  liberante nell'orizzonte - VEH 2
    % ========================================================

    for kk = 2:N+1

        if pos_hor_tail_2(kk) >= s_light
            i_tail_cross = kk;
            break
        end

    end

    if i_tail_cross == 0

        main_case = 5;

        if x_TL(1,ii) == 1

            current_green_end = local_current_green_end(x_TL, ii, N);

            if current_green_end > 0

                tail_at_green_end = pos_hor_tail_2(current_green_end);

                % ====================================================
                % Stima cinematica conservativa clearing coda - VEH 2
                % ====================================================

                dist_tail_to_TL = s_light - pos_hor_tail_2(1);

                if dist_tail_to_TL < 0
                    dist_tail_to_TL = 0;
                end

                v0_clear = vel_hor_2(1);

                if v0_clear < 0
                    v0_clear = 0;
                end

                a_clear     = 0.7;      % [m/s^2]
                v_max_clear = Vmax_2;   % [m/s]

                if dist_tail_to_TL <= 0

                    t_clear_tail = 0;

                else

                    if v0_clear >= v_max_clear || a_clear <= 0

                        t_clear_tail = dist_tail_to_TL / max(v0_clear, 0.1);

                    else

                        t_to_vmax = (v_max_clear - v0_clear) / a_clear;
                        d_to_vmax = v0_clear*t_to_vmax + 0.5*a_clear*t_to_vmax^2;

                        if dist_tail_to_TL <= d_to_vmax

                            t_clear_tail = ...
                                (-v0_clear + sqrt(v0_clear^2 + 2*a_clear*dist_tail_to_TL)) / a_clear;

                        else

                            t_clear_tail = ...
                                t_to_vmax + (dist_tail_to_TL - d_to_vmax) / v_max_clear;

                        end

                    end

                end

                dt_pred = 1.0;
                kk_tail_clear_est = ceil(t_clear_tail/dt_pred) + 1;

                if kk_tail_clear_est < 2
                    kk_tail_clear_est = 2;
                end

                tail_margin_nodes = 1;

                % ====================================================
                % CASE 8 - Fallback cinematico positivo - VEH 2
                % ====================================================

                if kk_tail_clear_est + tail_margin_nodes <= current_green_end

                    for kk = 2:N+1

                        idx_head = idx_head0_2 + ii + N_od*(kk-1);
                        idx_tail = idx_tail0_2 + ii + N_od*(kk-1);

                        OnlineData(idx_head) = 1;

                        if kk < kk_tail_clear_est
                            OnlineData(idx_tail) = 0;
                        else
                            OnlineData(idx_tail) = 1;
                        end

                    end

                    main_case       = 8;
                    green_window_ok = 1;

                    debug_TL_2(ii,:) = local_debug_row_veh( ...
                        time_cur, ii, s_light, ...
                        pos_hor_2, pos_hor_tail_2, vel_hor_2, ...
                        reached_TL_old_2, reached_TL_2, x_TL, OnlineData, ...
                        N_od, idx_head0_2, idx_tail0_2, ...
                        head_crossed_now_2, tail_crossed_now_2, head_stopped_at_light_2, ...
                        mem_case, main_case, current_green_end, ...
                        i_head_cross, i_tail_cross, green_window_ok, tail_at_green_end);

                    continue

                else

                    d_avail     = s_light - pos_hor_2(1);
                    d_stop_phys = vel_hor_2(1)^2/(2*a_brake_guard);

                    already_stopped_before_line = ...
                        (vel_hor_2(1) <= v_stop_thr_guard) && (d_avail >= 0);

                    can_still_stop = ...
                        already_stopped_before_line || ...
                        (d_avail >= d_stop_phys + d_margin_guard);

                    stopline_green_release = ...
                        (x_TL(1,ii) == 1) && ...
                        (d_avail >= 0) && ...
                        (d_avail <= eps_line) && ...
                        (vel_hor_2(1) <= v_stop_thr_guard);

                    if stopline_green_release
                    
                        % =================================================
                        % CASE 9A - GREEN COMMIT DA STOP-LINE - VEH 2
                        % =================================================
                    
                        for kk_case9 = 1:N+1
                    
                            idx_head = idx_head0_2 + ii + N_od*(kk_case9-1);
                            idx_tail = idx_tail0_2 + ii + N_od*(kk_case9-1);
                    
                            OnlineData(idx_head) = 1;
                            OnlineData(idx_tail) = 1;
                    
                        end
                    
                        reached_TL_2(ii) = 1;
                        mem_case         = 4;     % green commit
                        main_case        = 9;
                        green_window_ok  = 1;
                    
                        debug_TL_2(ii,:) = local_debug_row_veh( ...
                            time_cur, ii, s_light, ...
                            pos_hor_2, pos_hor_tail_2, vel_hor_2, ...
                            reached_TL_old_2, reached_TL_2, x_TL, OnlineData, ...
                            N_od, idx_head0_2, idx_tail0_2, ...
                            head_crossed_now_2, tail_crossed_now_2, head_stopped_at_light_2, ...
                            mem_case, main_case, current_green_end, ...
                            i_head_cross, i_tail_cross, green_window_ok, tail_at_green_end);
                    
                        continue

                    elseif can_still_stop || d_avail >= eps_line

                        % =============================================
                        % CASE 9B - Blocco ingresso - VEH 2
                        % =============================================

                        for kk_case9 = 2:current_green_end

                            idx_head = idx_head0_2 + ii + N_od*(kk_case9-1);
                            idx_tail = idx_tail0_2 + ii + N_od*(kk_case9-1);

                            OnlineData(idx_head) = 0;
                            OnlineData(idx_tail) = 0;

                        end

                        main_case = 9.3;

                    end

                    green_window_ok = 0;

                    debug_TL_2(ii,:) = local_debug_row_veh( ...
                        time_cur, ii, s_light, ...
                        pos_hor_2, pos_hor_tail_2, vel_hor_2, ...
                        reached_TL_old_2, reached_TL_2, x_TL, OnlineData, ...
                        N_od, idx_head0_2, idx_tail0_2, ...
                        head_crossed_now_2, tail_crossed_now_2, head_stopped_at_light_2, ...
                        mem_case, main_case, current_green_end, ...
                        i_head_cross, i_tail_cross, green_window_ok, tail_at_green_end);

                    continue

                end

            end

        end

        % ====================================================
        % CASE 5 - Default con coda non attraversante - VEH 2
        % ====================================================

        d_avail = s_light - pos_hor_2(1);

        case5_crossed = d_avail < -eps_cross_now;

        if case5_crossed

            for kk_case5 = 1:N+1

                idx_head = idx_head0_2 + ii + N_od*(kk_case5-1);
                idx_tail = idx_tail0_2 + ii + N_od*(kk_case5-1);

                OnlineData(idx_head) = 1;
                OnlineData(idx_tail) = 1;

            end

            reached_TL_2(ii) = 1;
            main_case = 10;
            mem_case  = 2;

        end

        debug_TL_2(ii,:) = local_debug_row_veh( ...
            time_cur, ii, s_light, ...
            pos_hor_2, pos_hor_tail_2, vel_hor_2, ...
            reached_TL_old_2, reached_TL_2, x_TL, OnlineData, ...
            N_od, idx_head0_2, idx_tail0_2, ...
            head_crossed_now_2, tail_crossed_now_2, head_stopped_at_light_2, ...
            mem_case, main_case, current_green_end, ...
            i_head_cross, i_tail_cross, green_window_ok, tail_at_green_end);

        continue

    end

    % ========================================================
    % Verifica finestra verde comune testa/coda - VEH 2
    % ========================================================

    green_info = local_find_green_window_vec(x_TL, ii, N, i_head_cross, i_tail_cross);

    green_window_ok = green_info(1);
    green_start     = green_info(2);
    green_end       = green_info(3);

    if green_window_ok == 1

        release_head_from = i_head_cross;
        release_tail_from = i_tail_cross;

        if green_start > 1

            if x_TL(green_start-1,ii) == 0 && x_TL(green_start,ii) == 1

                release_head_from = max(release_head_from, green_start);
                release_tail_from = max(release_tail_from, green_start);

            end

        end

        if release_head_from > green_end || release_tail_from > green_end

            main_case       = 7;
            green_window_ok = 0;

        else

            % =================================================
            % CASE 6 - Attraversamento valido stessa finestra verde - VEH 2
            % =================================================

            for kk = 2:N+1

                idx_head = idx_head0_2 + ii + N_od*(kk-1);
                idx_tail = idx_tail0_2 + ii + N_od*(kk-1);

                if kk < release_head_from
                    OnlineData(idx_head) = 0;
                else
                    OnlineData(idx_head) = 1;
                end

                if kk < release_tail_from
                    OnlineData(idx_tail) = 0;
                else
                    OnlineData(idx_tail) = 1;
                end

            end

            main_case = 6;

        end

    else

        main_case = 7;

    end

    % ========================================================
    % PROTEZIONE AGGIUNTIVA CASE 7 SU VERDE CORRENTE - VEH 2
    % ========================================================

    if main_case == 7 && x_TL(1,ii) == 1

        current_green_end = local_current_green_end(x_TL, ii, N);

        if current_green_end > 0

            d_avail     = s_light - pos_hor_2(1);
            d_stop_phys = vel_hor_2(1)^2/(2*a_brake_guard);

            already_stopped_before_line = ...
                (vel_hor_2(1) <= v_stop_thr_guard) && (d_avail >= 0);

            can_still_stop = ...
                already_stopped_before_line || ...
                (d_avail >= d_stop_phys + d_margin_guard);

            stopline_green_release = ...
                (x_TL(1,ii) == 1) && ...
                (d_avail >= 0) && ...
                (d_avail <= eps_line) && ...
                (vel_hor_2(1) <= v_stop_thr_guard);

            if stopline_green_release

                % ====================================================
                % CASE 7A - GREEN COMMIT DA STOP-LINE - VEH 2
                % ====================================================
            
                for kk_case7 = 1:N+1
            
                    idx_head = idx_head0_2 + ii + N_od*(kk_case7-1);
                    idx_tail = idx_tail0_2 + ii + N_od*(kk_case7-1);
            
                    OnlineData(idx_head) = 1;
                    OnlineData(idx_tail) = 1;
            
                end
            
                reached_TL_2(ii) = 1;
                mem_case         = 4;     % green commit
                main_case        = 7.3;
                green_window_ok  = 1;
            
            elseif can_still_stop || d_avail >= eps_line

                % ====================================================
                % CASE 7B - Blocco ingresso - VEH 2
                % ====================================================

                for kk_case7 = 2:current_green_end

                    idx_head = idx_head0_2 + ii + N_od*(kk_case7-1);
                    idx_tail = idx_tail0_2 + ii + N_od*(kk_case7-1);

                    OnlineData(idx_head) = 0;
                    OnlineData(idx_tail) = 0;

                end

                green_window_ok = 0;
                main_case = 7.6;

            end

        end

    end

    % ========================================================
    % DEBUG FINALE SEMAFORO ii - VEH 2
    % ========================================================

    debug_TL_2(ii,:) = local_debug_row_veh( ...
        time_cur, ii, s_light, ...
        pos_hor_2, pos_hor_tail_2, vel_hor_2, ...
        reached_TL_old_2, reached_TL_2, x_TL, OnlineData, ...
        N_od, idx_head0_2, idx_tail0_2, ...
        head_crossed_now_2, tail_crossed_now_2, head_stopped_at_light_2, ...
        mem_case, main_case, current_green_end, ...
        i_head_cross, i_tail_cross, green_window_ok, tail_at_green_end);

end






end




% ============================================================
% LOCAL DEBUG ROW GENERICA CON OFFSET TESTA/CODA
% ============================================================
function row = local_debug_row_veh(time_cur, ii, s_light, pos_hor, pos_hor_tail, vel_hor, ...
    reached_TL_old, reached_TL, x_TL, OnlineData, N_od, idx_head0, idx_tail0, ...
    head_crossed_now, tail_crossed_now, head_stopped_at_light, ...
    mem_case, main_case, current_green_end, i_head_cross, i_tail_cross, ...
    green_window_ok, tail_at_green_end)

row = zeros(1,26);

idx_head_k1 = idx_head0 + ii;
idx_tail_k1 = idx_tail0 + ii;

idx_head_k2 = idx_head0 + ii + N_od;
idx_tail_k2 = idx_tail0 + ii + N_od;

row(1)  = time_cur;
row(2)  = ii;
row(3)  = s_light;
row(4)  = pos_hor(1);
row(5)  = vel_hor(1);
row(6)  = pos_hor_tail(1);

row(7)  = reached_TL_old(ii);
row(8)  = reached_TL(ii);

row(9)  = x_TL(1,ii);
row(10) = x_TL(2,ii);
row(11) = x_TL(3,ii);

row(12) = double(head_crossed_now);
row(13) = double(tail_crossed_now);
row(14) = double(head_stopped_at_light);

row(15) = mem_case;
row(16) = main_case;

row(17) = current_green_end;
row(18) = i_head_cross;
row(19) = i_tail_cross;
row(20) = green_window_ok;
row(21) = tail_at_green_end;

row(22) = OnlineData(idx_head_k1);
row(23) = OnlineData(idx_tail_k1);
row(24) = OnlineData(idx_head_k2);
row(25) = OnlineData(idx_tail_k2);

row(26) = s_light - pos_hor(1);

end



% ============================================================
% LOCAL FUNCTION: LOCAL FIND GREEN WINDOW
% ============================================================
function green_info = local_find_green_window_vec(x_TL, ii, N, i_head_cross, i_tail_cross)

green_window_ok = 0;
green_start = 0;
green_end = 0;

kk = 1;

while kk <= N + 1

    if x_TL(kk,ii) == 1

        run_start = kk;

        while kk <= N + 1 && x_TL(kk,ii) == 1
            kk = kk + 1;
        end

        run_end = kk - 1;

        if i_head_cross >= run_start && i_tail_cross <= run_end
            green_window_ok = 1;
            green_start = run_start;
            green_end = run_end;
            break
        end

    else
        kk = kk + 1;
    end
end

green_info = zeros(1,3);
green_info(1) = green_window_ok;
green_info(2) = green_start;
green_info(3) = green_end;

end



% ============================================================
% LOCAL FUNCTION: CURRENT GREEN WINDOW END
% ============================================================
function green_end = local_current_green_end(x_TL, ii, N)

green_end = 0;

if x_TL(1,ii) == 0
    return
end

kk = 1;

while kk <= N+1 && x_TL(kk,ii) == 1
    green_end = kk;
    kk = kk + 1;
end

end




%debug function:
function row = local_debug_row(time_cur, ii, s_light, pos_hor, pos_hor_tail, vel_hor, ...
    reached_TL_old, reached_TL, x_TL, OnlineData, N_od, idx_tail0, ...
    head_crossed_now, tail_crossed_now, head_stopped_at_light, ...
    mem_case, main_case, current_green_end, i_head_cross, i_tail_cross, ...
    green_window_ok, tail_at_green_end)

row = zeros(1,26);

idx_head_k1 = ii;
idx_tail_k1 = idx_tail0 + ii;

idx_head_k2 = ii + N_od;
idx_tail_k2 = idx_tail0 + ii + N_od;

idx_head_k3 = ii + 2*N_od;
idx_tail_k3 = idx_tail0 + ii + 2*N_od;

idx_head_k4 = ii + 3*N_od;
idx_tail_k4 = idx_tail0 + ii + 3*N_od;

idx_head_k5 = ii + 4*N_od;
idx_tail_k5 = idx_tail0 + ii + 4*N_od;

row(1)  = time_cur;
row(2)  = ii;
row(3)  = s_light;
row(4)  = pos_hor(1);
row(5)  = vel_hor(1);
row(6)  = pos_hor_tail(1);

row(7)  = reached_TL_old(ii);
row(8)  = reached_TL(ii);

row(9)  = x_TL(1,ii);
row(10) = x_TL(2,ii);
row(11) = x_TL(3,ii);

row(12) = double(head_crossed_now);
row(13) = double(tail_crossed_now);
row(14) = double(head_stopped_at_light);

row(15) = mem_case;
row(16) = main_case;

row(17) = current_green_end;
row(18) = i_head_cross;
row(19) = i_tail_cross;
row(20) = green_window_ok;
row(21) = tail_at_green_end;

row(22) = OnlineData(idx_head_k1);
row(23) = OnlineData(idx_tail_k1);
row(24) = OnlineData(idx_head_k2);
row(25) = OnlineData(idx_tail_k2);

row(26) = s_light - pos_hor(1);

end
